simulink model "raspberrypi_multicore_audio"  (R2021b)
settings: Solver=VariableStepAuto  StartTime=0.0  StopTime=10.0  RelTol=1e-3
undefined symbols (not defined in the file): plughw
libraries: audiofilters x3, raspberrypiAVlib x2, audiodynamicrange x1, dspindex x1
settings Model: Creator=The MathWorks, Inc.  LastModifiedBy=The MathWorks, Inc.
settings SolverCC: AlgebraicLoopSolver=TrustRegion
settings DebuggingCC: SFMachineParentedDataDiag=warning

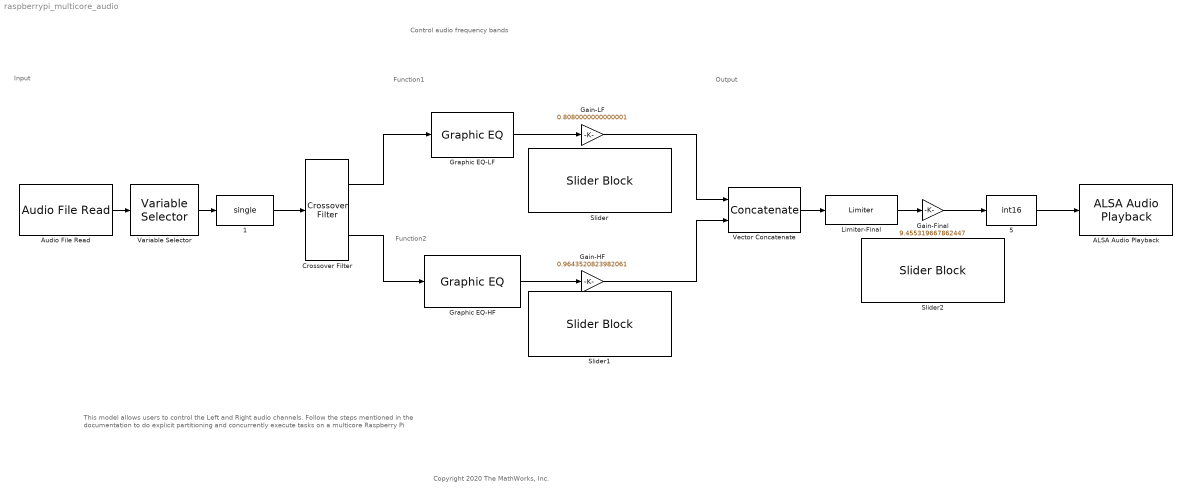
== system raspberrypi_multicore_audio ==
  note: Output
  note: Function1
  note: Input
  note: Control audio frequency bands
  note: Copyright 2020 The MathWorks, Inc.
  note: Function2
  note: This model allows users to control the Left and Right audio channels. Follow the steps mentioned in the documentation to do explicit partitioning and concurrently execute tasks on a multicore Raspberry Pi
  " 1" : DataTypeConversion  OutDataTypeStr=single
  " 5" : DataTypeConversion  OutDataTypeStr=int16
  ALSA Audio Playback : raspberrypiAVlib/ALSA Audio Playback  deviceStr=plughw:1,0  sampleRateEnum=44100  queueDuration=0.5  blockPlatform=RASPBERRYPI
      settings: SourceProductBaseCode=RASPPI
  Audio File Read : raspberrypiAVlib/Audio File Read  FileName=guitartune.wav  PlayCount=Inf  OutputEOFIndicator=off  SamplesPerFrame=4410
      settings: SourceProductBaseCode=RASPPI
  Crossover Filter : audiofilters/Crossover Filter  NCrossovers=1  Crossover1Port=off  Crossover1=2.218e+03  Order1Port=off  Order1=8  Crossover2Port=off  Crossover2=800  Order2Port=off  Order2=2  Crossover3Port=off  Crossover3=1500  Order3Port=off  Order3=2  Crossover4Port=off  Crossover4=3000  Order4Port=off  Order4=2  InheritSampleRate=off  SampleRate=44100  SimulateUsing=Code generation
      settings: SourceProductBaseCode=AU
  Gain-Final : Gain  Gain=9.455319667862447  OutDataTypeStr=int16
  Gain-HF : Gain  Gain=0.9643520823982061  OutDataTypeStr=single
  Gain-LF : Gain  Gain=0.8080000000000001  OutDataTypeStr=single
  Graphic EQ-HF : audiofilters/Graphic EQ  EQOrder=2  Bandwidth=2/3 octave  Structure=Cascade  Gain_25=-20  Gain_31_5=-20  Gain_40=-20  Gain_50=0  Gain_63=-20  Gain_80=0  Gain_100=-20  Gain_125=-20  Gain_160=-20  Gain_200=0  Gain_250=-20  Gain_315=-1.200  Gain_400=-20  Gain_500=6  Gain_630=-20  Gain_800=0  Gain_1000=0  Gain_1250=0  Gain_1600=3  Gain_2000=6  Gain_2500=3  Gain_3150=0  Gain_4000=0.0  Gain_5000=0  Gain_6300=6  Gain_8000=12  Gain_10000=6  Gain_12500=0  Gain_16000=6  Gain_20000=0  InheritSampleRate=off  SampleRate=44100  SimulateUsing=Code generation
      settings: SourceProductBaseCode=AU
  Graphic EQ-LF : audiofilters/Graphic EQ  EQOrder=2  Bandwidth=2/3 octave  Structure=Cascade  Gain_25=12  Gain_31_5=16  Gain_40=16  Gain_50=0  Gain_63=12  Gain_80=0  Gain_100=12  Gain_125=16  Gain_160=12  Gain_200=0  Gain_250=12  Gain_315=-1.200  Gain_400=10.800  Gain_500=6  Gain_630=6  Gain_800=0  Gain_1000=5  Gain_1250=0  Gain_1600=6  Gain_2000=6  Gain_2500=6  Gain_3150=0  Gain_4000=-20  Gain_5000=0  Gain_6300=-20  Gain_8000=-20  Gain_10000=-20  Gain_12500=0  Gain_16000=-20  Gain_20000=0  InheritSampleRate=off  SampleRate=44100  SimulateUsing=Code generation
      settings: SourceProductBaseCode=AU
  Limiter-Final : audiodynamicrange/Limiter  ThresholdPort=off  Threshold=-8.0  KneeWidthPort=off  KneeWidth=17.600  AttackTimePort=off  AttackTime=0.9995  ReleaseTimePort=off  ReleaseTime=0.0005  MakeUpGainMode=Property  MakeUpGain=10  InheritSampleRate=off  SampleRate=44100  outputGain=off  EnableSidechain=off  SimulateUsing=Code generation
      settings: SourceProductBaseCode=AU
  Slider : SliderBlock  LabelPosition=Bottom  ScaleMax=1
  Slider1 : SliderBlock  LabelPosition=Bottom  ScaleMax=1
  Slider2 : SliderBlock  LabelPosition=Bottom  ScaleMax=10
  Variable Selector : dspindex/Variable Selector  NumInputs=1  rowsOrCols=Columns  IdxMode=Fixed  Elements=1  ZerOneIdxMode=One-based  errmode=Clip Index  FillMode=on  FillValues=0
  Vector Concatenate : Concatenate  Mode=Multidimensional array  ConcatenateDimension=2
  wires:
  Audio File Read/1 -> Variable Selector/1
  " 1"/1 -> Crossover Filter/1
  Variable Selector/1 -> " 1"/1
  Crossover Filter/1 -> Graphic EQ-LF/1
  Crossover Filter/2 -> Graphic EQ-HF/1
  Graphic EQ-LF/1 -> Gain-LF/1
  Graphic EQ-HF/1 -> Gain-HF/1
  Limiter-Final/1 -> Gain-Final/1
  " 5"/1 -> ALSA Audio Playback/1
  Gain-LF/1 -> Vector Concatenate/1
  Vector Concatenate/1 -> Limiter-Final/1
  Gain-HF/1 -> Vector Concatenate/2
  Gain-Final/1 -> " 5"/1
